simulink model "LQG"  (R2021b)
settings: Solver=VariableStepAuto  StartTime=0.0  StopTime=100  RelTol=1e-3
libraries: cstblocks x1
settings Model: Creator=hongp  LastModifiedBy=hongp

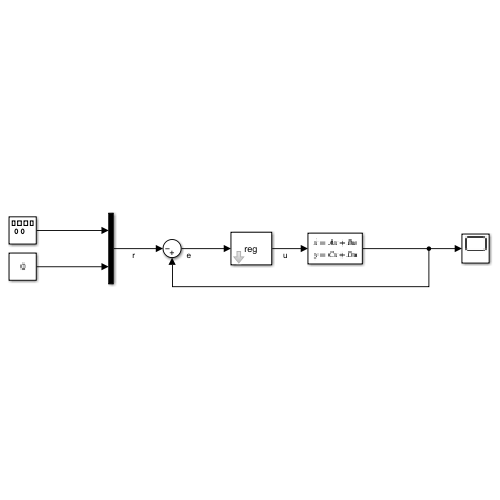
[thumbnail: Simulink's stored preview of the top-level diagram]
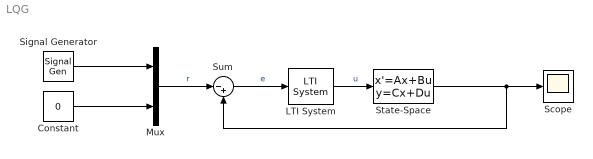
== system LQG ==
  Constant : Constant  Value=0
  LTI System : cstblocks/LTI System  sys=reg  IC=[]
  Mux : Mux  Inputs=2
  Scope : Scope
  Signal Generator : SignalGenerator  WaveForm=square  Amplitude=pi/2  Frequency=0.1  Units=rad/sec
  State-Space : StateSpace  A=[0 0 1 0;0 0 0 1;0 149.3 -0.01 0;0 261.6 -0.01 0]  B=[0;0;49.73;49.73]  C=[1 0 0 0;0 1 0 0]  D=[0;0]  InitialCondition=0
  Sum : Sum  Inputs=|-+
  wires:
  Constant/1 -> Mux/2
  LTI System/1 -> State-Space/1  "u"
  Sum/1 -> LTI System/1  "e"
  State-Space/1 -> Sum/2, Scope/1
  Mux/1 -> Sum/1  "r"
  Signal Generator/1 -> Mux/1
